simulink model "Copy_of_PositionBlockDiagram"  (R2020a)
settings: Solver=VariableStepAuto  StartTime=0.0  StopTime=16  RelTol=1e-3
undefined symbols (not defined in the file): DiscIntNeverNeededParam
libraries: simulink x1
settings Model: Creator=scott  LastModifiedBy=scott

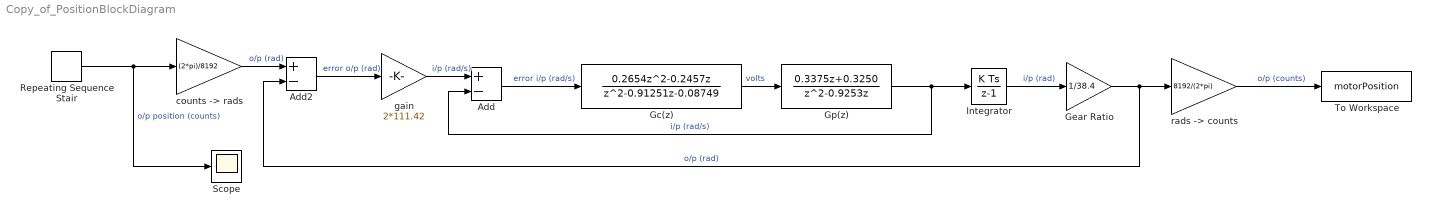
== system Copy_of_PositionBlockDiagram ==
  Add : Sum  Inputs=+-
  Add2 : Sum  Inputs=+-
  Gc(z) : DiscreteTransferFcn  Numerator=[0.2654 -0.2457 0]  Denominator=[1 -0.91251 -0.08749]  SampleTime=0.008
  Gear Ratio : Gain  Gain=1/38.4
  Gp(z) : DiscreteTransferFcn  Numerator=[0.3375 0.3250]  Denominator=[1 -0.9253 0]  SampleTime=0.008
  Integrator : DiscreteIntegrator  SampleTime=0.008  ICPrevOutput=DiscIntNeverNeededParam  ICPrevScaledInput=DiscIntNeverNeededParam
  Repeating Sequence Stair : simulink/Sources/Repeating Sequence Stair  OutValues=[3072 1024 2048 2560 0].'  tsamp=3.2  OutMin=[]  OutMax=[]  OutDataTypeStr=double  OutputDataTypeScalingMode=double  OutDataType=fixdt(0,8)  ConRadixGroup=Best Precision: Vector-wise  OutScaling=2^-12
  Scope : Scope
  To Workspace : ToWorkspace  VariableName=motorPosition  SaveFormat=Timeseries  SampleTime=-1
  "counts -> rads" : Gain  Gain=(2*pi)/8192
  gain : Gain  Gain=2*111.42
  "rads -> counts" : Gain  Gain=8192/(2*pi)
  wires:
  "rads -> counts"/1 -> To Workspace/1  "o/p (counts)"
  Add2/1 -> gain/1  "error o/p (rad)"
  gain/1 -> Add/1  "i/p (rad/s)"
  Add/1 -> Gc(z)/1  "error i/p (rad/s)"
  Integrator/1 -> Gear Ratio/1  "i/p (rad)"
  Gear Ratio/1 -> Add2/2, "rads -> counts"/1  "o/p (rad)"
  Gc(z)/1 -> Gp(z)/1  "volts"
  Repeating Sequence Stair/1 -> "counts -> rads"/1, Scope/1  "o/p position (counts)"
  "counts -> rads"/1 -> Add2/1  "o/p (rad)"
  Gp(z)/1 -> Integrator/1, Add/2  "i/p (rad/s)"
